simulink model "pid_and_lag"  (R2022b)
settings: Solver=VariableStepAuto  StartTime=0.0  StopTime=10.0  RelTol=1e-3
undefined symbols (not defined in the file): Kd, Ki, Kp, N
settings Model: Creator=saayu  LastModifiedBy=saayu

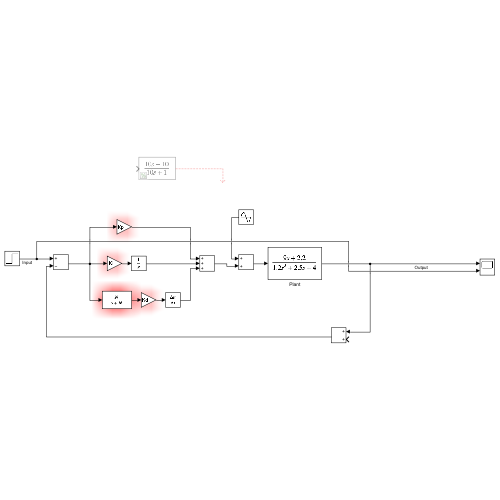
[thumbnail: Simulink's stored preview of the top-level diagram]
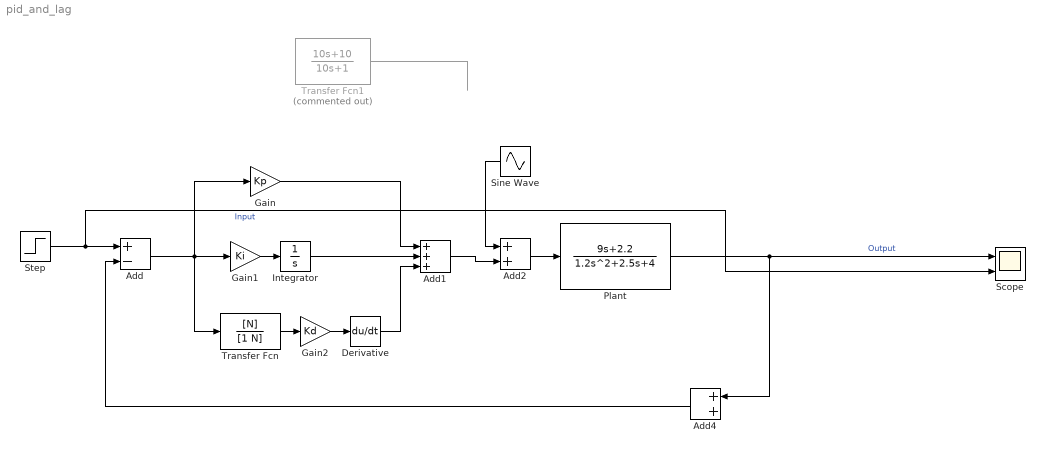
== system pid_and_lag ==
  Add : Sum  Inputs=+-
  Add1 : Sum  Inputs=+++
  Add2 : Sum
  Add4 : Sum
  Derivative : Derivative
  Gain : Gain  Gain=Kp
  Gain1 : Gain  Gain=Ki
  Gain2 : Gain  Gain=Kd
  Integrator : Integrator
  Plant : TransferFcn  Numerator=[9 2.2]  Denominator=[1.2 2.5 4]
  Scope : Scope  NumInputPorts=2
  Sine Wave : Sin  SampleTime=0
  Step : Step  SampleTime=0
  Transfer Fcn : TransferFcn  Numerator=[N]  Denominator=[1 N]
  Transfer Fcn1 : TransferFcn  Commented=on  Numerator=[10 10]  Denominator=[10 1]
  wires:
  Add/1 -> Transfer Fcn/1, Gain/1, Gain1/1
  Add1/1 -> Add2/2
  Derivative/1 -> Add1/3
  Transfer Fcn/1 -> Gain2/1
  Add4/1 -> Add/2
  Gain2/1 -> Derivative/1
  Gain/1 -> Add1/1
  Gain1/1 -> Integrator/1
  Integrator/1 -> Add1/2
  Plant/1 -> Add4/1, Scope/1  "Output"
  Step/1 -> Scope/2, Add/1  "Input"
  Add2/1 -> Plant/1
  Sine Wave/1 -> Add2/1
  Transfer Fcn1/1 -> ?
